simulink model "Proj_P1"  (R2020a)
settings: Solver=VariableStepAuto  StartTime=0.0  StopTime=10.0  RelTol=1e-3
undefined symbols (not defined in the file): Kp
settings Model: Creator=jguil  LastModifiedBy=jguil

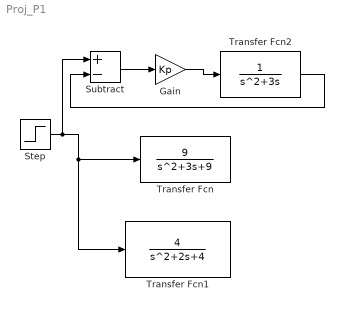
== system Proj_P1 ==
  Gain : Gain  Gain=Kp
  Step : Step  SampleTime=0
  Subtract : Sum  Inputs=+-
  Transfer Fcn : TransferFcn  Numerator=[9]  Denominator=[1 3 9]
  Transfer Fcn1 : TransferFcn  Numerator=[4]  Denominator=[1 2 4]
  Transfer Fcn2 : TransferFcn  Denominator=[1 3 0]
  wires:
  Gain/1 -> Transfer Fcn2/1
  Subtract/1 -> Gain/1
  Step/1 -> Subtract/1, Transfer Fcn1/1, Transfer Fcn/1
  Transfer Fcn2/1 -> Subtract/2
